simulink model "Diagrama_de_fase"  (R2017a)
settings: Solver=VariableStepAuto  StartTime=0.0  StopTime=10.0  RelTol=1e-3
values from neighbouring files (symbols this model uses):
  a11 = 1    [Diagrama_de_faseM.m]
  a12 = 0    [Diagrama_de_faseM.m]
  a21 = 0    [Diagrama_de_faseM.m]
  a22 = 2    [Diagrama_de_faseM.m]
libraries: simulink x1
settings Model: Creator=franj  LastModifiedBy=franj

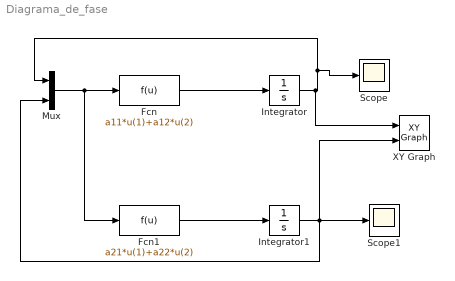
== system Diagrama_de_fase ==
  Fcn : Fcn  Expr=a11*u(1)+a12*u(2)
  Fcn1 : Fcn  Expr=a21*u(1)+a22*u(2)
  Integrator : Integrator  InitialCondition=1.5
  Integrator1 : Integrator  InitialCondition=2
  Mux : Mux  Inputs=2
  Scope : Scope
  Scope1 : Scope
  XY Graph : simulink/Sinks/XY Graph  xmin=-1  xmax=1  ymin=-1  ymax=1  st=-1
  wires:
  Mux/1 -> Fcn1/1, Fcn/1
  Integrator/1 -> XY Graph/1, Scope/1, Mux/1
  Fcn/1 -> Integrator/1
  Fcn1/1 -> Integrator1/1
  Integrator1/1 -> XY Graph/2, Scope1/1, Mux/2
